simulink model "Parcial3_adquisicion_Datos"  (R2016a)
settings: Solver=VariableStepAuto  StartTime=0.0  StopTime=1500  RelTol=1e-3
values from neighbouring files (symbols this model uses):
  tm = 0.1    [ejemplodiscretro.m]
undefined symbols (not defined in the file or in its folder): ts
settings Model: Creator=Daniel  LastModifiedBy=Daniel

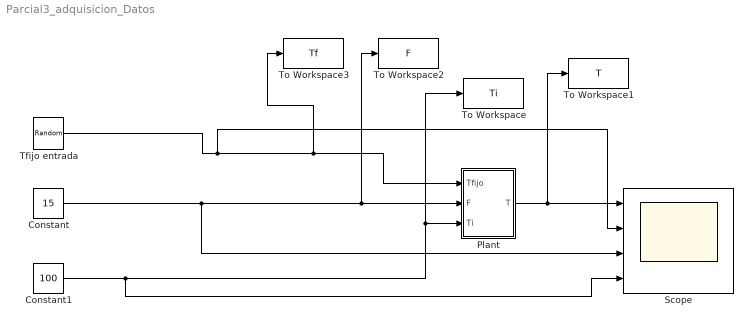
== system Parcial3_adquisicion_Datos ==
  Constant : Constant  Value=15
  Constant1 : Constant  Value=100
  Plant : Subsystem
  Scope : Scope  NumInputPorts=4
  Tfijo entrada : UniformRandomNumber  Minimum=130  Maximum=170  SampleTime=ts
  To Workspace : ToWorkspace  VariableName=Ti  SampleTime=tm
  To Workspace1 : ToWorkspace  VariableName=T  SampleTime=tm
  To Workspace2 : ToWorkspace  VariableName=F  SampleTime=tm
  To Workspace3 : ToWorkspace  VariableName=Tf  SampleTime=tm
  wires:
  Plant/1(T) -> Scope/1, To Workspace1/1
  Constant/1 -> To Workspace2/1, Plant/2(F), Scope/3
  Constant1/1 -> To Workspace/1, Plant/3(Ti), Scope/4
  Tfijo entrada/1 -> To Workspace3/1, Plant/1(Tfijo), Scope/2

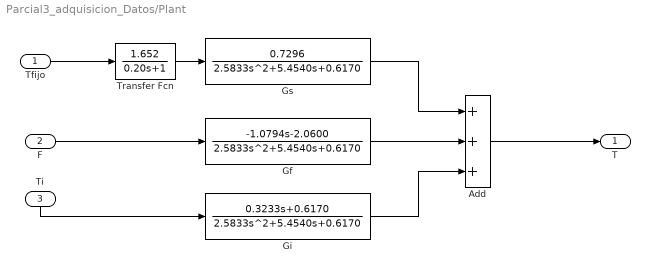
== system Parcial3_adquisicion_Datos/Plant ==
  Tfijo : Inport
  F : Inport  Port=2
  Ti : Inport  Port=3
  Add : Sum  Inputs=+++
  Gf : TransferFcn  Numerator=[-1.0794 -2.0600]  Denominator=[2.5833 5.4540 0.6170]
  Gi : TransferFcn  Numerator=[0.3233 0.6170]  Denominator="[2.5833 5.4540  0.6170]"
  Gs : TransferFcn  Numerator=[0.7296]  Denominator="[2.5833 5.4540  0.6170]"
  Transfer Fcn : TransferFcn  Numerator=[1.652]  Denominator=[0.20 1]
  T : Outport
  wires:
  Add/1 -> T/1
  Gi/1 -> Add/3
  Gf/1 -> Add/2
  Transfer Fcn/1 -> Gs/1
  Gs/1 -> Add/1
  Ti/1 -> Gi/1
  Tfijo/1 -> Transfer Fcn/1
  F/1 -> Gf/1
